simulink model "test_pid"  (R2020b)
settings: Solver=VariableStepAuto  StartTime=0.0  StopTime=10.0  RelTol=1e-3
values from neighbouring files (symbols this model uses):
  Kd = 0    [ControllerModel_2020.m]
  Ki = 0.1    [ControllerModel_2020.m]
  Kp = 0.1    [ControllerModel_2020.m]
settings Model: Creator=005274  LastModifiedBy=005274

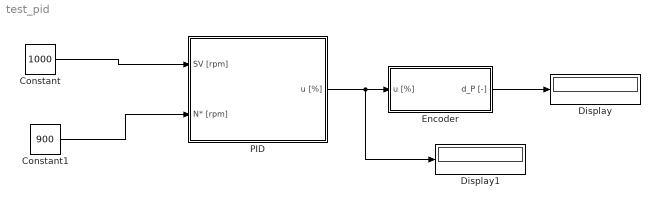
== system test_pid ==
  Constant : Constant  Value=1000
  Constant1 : Constant  Value=900
  Display : Display
  Display1 : Display
  Encoder : Subsystem  mask{n=8}
      mask prompts: n "bit"
  PID : Subsystem
  wires:
  Constant1/1 -> PID/2(N* [rpm])
  Constant/1 -> PID/1(SV [rpm])
  PID/1(u [%]) -> Display1/1, Encoder/1(u [%])
  Encoder/1(d_P [-]) -> Display/1

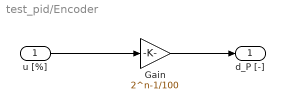
== system test_pid/Encoder ==
  u [%] : Inport
  Gain : Gain  Gain=2^n-1/100
  d_P [-] : Outport
  wires:
  Gain/1 -> d_P [-]/1
  u [%]/1 -> Gain/1

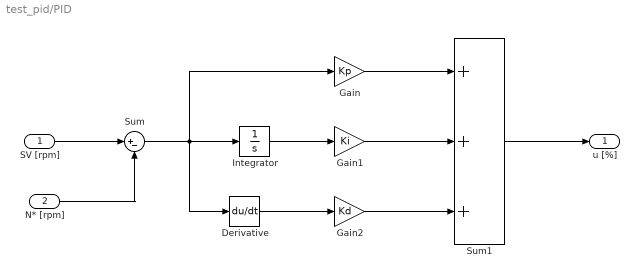
== system test_pid/PID ==
  SV [rpm] : Inport
  N* [rpm] : Inport  Port=2
  Derivative : Derivative
  Gain : Gain  Gain=Kp
  Gain1 : Gain  Gain=Ki
  Gain2 : Gain  Gain=Kd
  Integrator : Integrator
  Sum : Sum  Inputs=|+-
  Sum1 : Sum  Inputs=+++
  u [%] : Outport
  wires:
  N* [rpm]/1 -> Sum/2
  SV [rpm]/1 -> Sum/1
  Sum/1 -> Derivative/1, Gain/1, Integrator/1
  Derivative/1 -> Gain2/1
  Integrator/1 -> Gain1/1
  Gain1/1 -> Sum1/2
  Gain/1 -> Sum1/1
  Gain2/1 -> Sum1/3
  Sum1/1 -> u [%]/1
